simulink model "pospoli_XY_traiettoria"  (R2020b)
settings: Solver=ode15s  StartTime=0.0  StopTime=tsim  MaxStep=0.024  RelTol=1e-3
values from neighbouring files (symbols this model uses):
  Acc_asse_x = []    [Main_Strategia_di_pilotaggio.m]
  Acc_asse_y = []    [Main_Strategia_di_pilotaggio.m]
  mx = config_dc_x(parx)    [Main_Strategia_di_pilotaggio.m]    (also in Main_traiettoria.m; Main_traiettoria_ordinato.m)
  my = config_dc_y(pary)    [Main_Strategia_di_pilotaggio.m]    (also in Main_traiettoria.m; Main_traiettoria_ordinato.m)
  ppx_c = pos_poli_cc_x(mx, acx, 2)    [Main_Strategia_di_pilotaggio.m]
  ppx_m = pos_poli_cc_x(mx, acx, 1)    [Main_Strategia_di_pilotaggio.m]
  ppy_c = pos_poli_cc_y(my, acy, 2)    [Main_Strategia_di_pilotaggio.m]
  ppy_m = pos_poli_cc_y(my, acy, 1)    [Main_Strategia_di_pilotaggio.m]
  time = 0:tf/np:tf    [Main_traiettoria.m]    (also in Main_traiettoria_ordinato.m = 0:passo:tsim)
  Vel_asse_x = []    [Main_Strategia_di_pilotaggio.m]
  Vel_asse_y = []    [Main_Strategia_di_pilotaggio.m]
  x = []    [Main_Strategia_di_pilotaggio.m]    (also in Main_traiettoria.m = zeros(length(time),1); Main_traiettoria_ordinato.m = zeros(length(time),1); interpolazione_tempi.m = interp1(t_m,x_i,u,'Linear'))
  y = []    [Main_Strategia_di_pilotaggio.m]    (also in Main_traiettoria.m = zeros(length(time),1); Main_traiettoria_ordinato.m = zeros(length(time),1); interpolazione_tempi.m = interp1(t_m,y_i,u,'Linear'))
undefined symbols (not defined in the file or in its folder): accelerazioni, accelerazioniy, ci_x, ci_y, Evaluate_Trajectory, interpolazione_tempi, parx, pary
libraries: simulink x2
settings Model: Creator=stefa  LastModifiedBy=user
settings DebuggingCC: AlgebraicLoopMsg=none  SFMachineParentedDataDiag=error

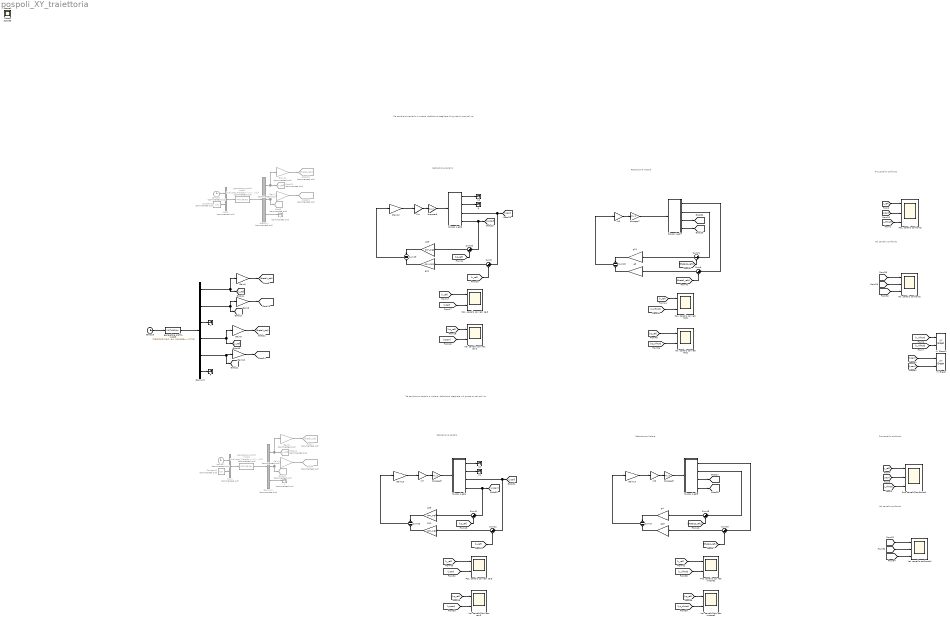
== system pospoli_XY_traiettoria ==
  note: Se cambiamo carrello o motore, dobbiamo scegliere w0 giusta su pos poli cc
  note: Retroazione Motore
  note: Se cambiamo carrello o motore, dobbiamo scegliere w0 giusta su pos poli cc
  note: Retroazione carrello
  note: Retroazione carrello
  note: Retroazione Motore
  note: Vel carrello confronto
  note: Pos carrello confronto
  note: Vel carrello confronto
  note: Pos carrello confronto
  " 1" : Terminator  Commented=on
   {7..12} (6 alike) : Terminator
  " 4" : Terminator  Commented=on
  Constant1 : Constant  Commented=on  Value=0.6
  Constant2 : Constant  Commented=on  Value=0.6
  Demux1 : Demux  Commented=on  Outputs=3
  Demux2 : Demux  Commented=on  Outputs=3
  Demux3 : Demux  Outputs=6
  Gain{9..10,13..14} (4 alike) : Gain  Gain=1/pary.tau
  Gain11 : Gain  Commented=on  Gain=1/parx.tau
  Gain12 : Gain  Gain=1/parx.tau
  Gain3 : Gain  Commented=on  Gain=1/pary.tau
  Gain4 : Gain  Commented=on  Gain=1/pary.tau
  Gain6 : Gain  Gain=1/parx.tau
  Gain7 : Gain  Commented=on  Gain=1/parx.tau
  Gain8 : Gain  Gain=1/parx.tau
  Goto10 : Goto  Commented=on  GotoTag=y_ref
  Goto11 : Goto  Commented=on  GotoTag=yp_ref
  Goto18 : Goto  Commented=on  GotoTag=theta1_refx
  Goto20 : Goto  Commented=on  GotoTag=theta1p_refx
  Goto23 : Goto  Commented=on  GotoTag=x_ref
  Goto5 : Goto  Commented=on  GotoTag=xp_ref
  Goto7 : Goto  Commented=on  GotoTag=theta1_refy
  Goto9 : Goto  Commented=on  GotoTag=theta1p_refy
  Kr4 : Gain  Gain=mx.Kr
  Kr6 : Gain  Gain=mx.Kr
  Kr7 : Gain  Gain=my.Kr
  Kr8 : Gain  Gain=my.Kr
  Mux1 : Mux  Commented=on  Inputs=2
  Mux2 : Mux  Commented=on  Inputs=2
  Pos. carrello con retr. Mot1 : Scope  NumInputPorts=2
  Pos. carrello con retr. car2 : Scope  NumInputPorts=2
  Pos. carrello con retr. car3 : Scope  NumInputPorts=2
  Pos. carrello con retr. motore1 : Scope  NumInputPorts=2
  Pos. carrello confronto : Scope  NumInputPorts=3
  Pos. carrello confronto1 : Scope  NumInputPorts=3
  Sum{6,8,11,15..16,20..22} (8 alike) : Sum  Inputs=|+-
  Sum{17..19,23} (4 alike) : Sum  Inputs=--
  Vel. carrello con retr. Mot1 : Scope  NumInputPorts=2
  Vel. carrello con retr. car.2 : Scope  NumInputPorts=2
  Vel. carrello con retr. car.3 : Scope  NumInputPorts=2
  Vel. carrello con retr. motore1 : Scope  NumInputPorts=2
  Vel. carrello confronto : Scope  NumInputPorts=3
  Vel. carrello confronto1 : Scope  NumInputPorts=3
  XY Graph : simulink/Sinks/XY Graph  xmin=-0.5  xmax=0.5  ymin=-0.5  ymax=0.5  st=-1
  XY Graph1 : simulink/Sinks/XY Graph  xmin=-0.5  xmax=0.5  ymin=-0.5  ymax=0.5  st=-1
  blocco 4 gdl4 : Subsystem
  blocco 4 gdl6 : Subsystem
  blocco 4 gdl7 : Subsystem
  blocco 4 gdl8 : Subsystem
  chopper3 : Gain  Gain=my.K
  chopper6 : Gain  Gain=mx.K
  chopper7 : Gain  Gain=mx.K
  chopper8 : Gain  Gain=my.K
  g11 : Gain  Gain=ppx_m.g2
  g12 : Gain  Gain=ppx_c.g1
  g13 : Gain  Gain=ppx_c.g2
  g14 : Gain  Gain=ppy_c.g1
  g15 : Gain  Gain=ppy_c.g2
  g16 : Gain  Gain=ppy_m.g1
  g3 : Gain  Gain=ppx_m.g1
  g4 : Gain  Gain=ppy_m.g2
  generatore profilo moto1 : MATLABFcn  Commented=on  MATLABFcn=Evaluate_Trajectory( u(1) , u(2))  OutputDimensions=3
  generatore profilo moto2 : MATLABFcn  Commented=on  MATLABFcn=Evaluate_Trajectory( u(1) , u(2))  OutputDimensions=3
  generatore profilo moto3 : MATLABFcn  MATLABFcn=interpolazione_tempi(x,Vel_asse_x,Acc_asse_x,y,Vel_asse_y,Acc_asse_y,u,time)
  tempo1 : Clock  Commented=on
  tempo2 : Clock  Commented=on
  tempo3 : Clock
      settings: Decimation=tsim
  Scope : Scope
  Scope1 : Scope
  Scope3 : Scope
  wires:
  Mux2/1 -> generatore profilo moto1/1
  Gain7/1 -> Goto20/1  "motore"
  Gain11/1 -> Goto18/1  "motore"
  Constant2/1 -> Mux2/2
  Demux1/3 -> " 1"/1  "XPP"
  tempo1/1 -> Mux2/1
  generatore profilo moto1/1 -> Demux1/1  "carrello"
  Demux1/2 -> Gain7/1, Goto5/1  "XP"
  Demux1/1 -> Goto23/1, Gain11/1  "X"
  tempo2/1 -> Mux1/1
  generatore profilo moto2/1 -> Demux2/1  "carrello"
  Demux2/2 -> Gain4/1, Goto11/1  "YP"
  Constant1/1 -> Mux1/2
  Mux1/1 -> generatore profilo moto2/1
  Gain4/1 -> Goto9/1  "motore"
  Gain3/1 -> Goto7/1  "motore"
  Demux2/1 -> Goto10/1, Gain3/1  "Y"
  Demux2/3 -> " 4"/1  "YPP"
  generatore profilo moto3/1 -> Demux3/1  "carrello"
  tempo3/1 -> generatore profilo moto3/1
  Demux3/6 -> " 8"/1  "YPP"
  Gain6/1 -> [theta1_refx]  "motore"
  Demux3/3 -> " 7"/1  "XPP"
  Demux3/1 -> [x_ref], Gain6/1  "X"
  Demux3/2 -> Gain8/1, [xp_ref]  "XP"
  Gain8/1 -> [theta1p_refx]  "motore"
  Gain9/1 -> [theta1_refy]  "motore"
  Gain10/1 -> [theta1p_refy]  "motore"
  Demux3/4 -> [y_ref], Gain9/1  "Y"
  Demux3/5 -> [yp_ref], Gain10/1  "YP"
  [x_rifmot] -> Pos. carrello con retr. Mot1/2  "motore"
  Kr7/1 -> chopper3/1  "I"
  Sum21/1 -> g11/1
  [theta1p_refx] -> Sum21/2
  Sum20/1 -> g13/1
  blocco 4 gdl7/1(Out3) -> Sum6/1
  g12/1 -> Sum19/2  "Cm"
  chopper6/1 -> blocco 4 gdl6/1(In1)  "Cm"
  chopper7/1 -> blocco 4 gdl7/1(In1)  "Cm"
  Sum6/1 -> g3/1
  g3/1 -> Sum18/2  "Cm"
  Sum18/1 -> Kr6/1  "Va"
  blocco 4 gdl7/4(Out1) -> [xp_rifmot]
  Kr6/1 -> chopper7/1  "I"
  g11/1 -> Sum18/1  "Cm"
  blocco 4 gdl8/4(Out1) -> [yp_rifmot]
  Gain14/1 -> Kr8/1  "motore"
  Sum16/1 -> g16/1
  blocco 4 gdl8/3(Out3) -> [y_rifmot]
  g4/1 -> Sum17/1  "Cm"
  [xcarr] -> Pos. carrello con retr. car2/2  "carrello"
  g15/1 -> Sum23/1  "Cm"
  Sum15/1 -> g4/1
  Kr8/1 -> chopper8/1  "I"
  blocco 4 gdl8/1(Out2) -> Sum16/1
  [theta1_refy] -> Sum16/2
  [yp_ref] -> Vel. carrello con retr. car.3/1
  g13/1 -> Sum19/1  "Cm"
  [theta1_refx] -> Sum6/2
  g14/1 -> Sum23/2  "Cm"
  blocco 4 gdl8/2(Out5) -> Sum15/1
  blocco 4 gdl4/3(Out3) -> Sum22/1, [ycarr]
  blocco 4 gdl6/1(Out3) -> " 10"/1
  [y_ref] -> Pos. carrello con retr. car3/1
  [x_ref] -> Sum8/2
  g16/1 -> Sum17/2  "Cm"
  blocco 4 gdl4/2(Out5) -> " 11"/1
  Sum22/1 -> g14/1
  blocco 4 gdl4/1(Out2) -> " 12"/1
  Kr4/1 -> chopper6/1  "I"
  blocco 4 gdl7/2(Out4) -> Sum21/1
  [xp_ref] -> Vel. carrello con retr. car.2/1
  Sum19/1 -> Gain12/1
  [yp_ref] -> Sum11/2
  blocco 4 gdl6/3(Out7) -> Sum8/1, [xcarr]
  blocco 4 gdl4/4(Out1) -> Sum11/1, [ypcarr]
  blocco 4 gdl6/2(Out4) -> " 9"/1
  Sum17/1 -> Gain14/1
  [ycarr] -> Pos. carrello con retr. car3/2  "carrello"
  [yp_ref] -> Vel. carrello con retr. motore1/1
  [x_ref] -> Pos. carrello con retr. car2/1
  chopper8/1 -> blocco 4 gdl8/1(In2)  "Cm"
  chopper3/1 -> blocco 4 gdl4/1(In2)  "Cm"
  Gain12/1 -> Kr4/1  "motore"
  [y_ref] -> Sum22/2
  [x_ref] -> Pos. carrello con retr. Mot1/1
  [xp_ref] -> Vel. carrello con retr. Mot1/1
  Sum23/1 -> Gain13/1
  [xp_rifmot] -> Vel. carrello con retr. Mot1/2  "motore"
  blocco 4 gdl7/3(Out7) -> [x_rifmot]
  [yp_rifmot] -> Vel. carrello con retr. motore1/2  "carrello"
  [theta1p_refy] -> Sum15/2
  blocco 4 gdl6/4(Out1) -> Sum20/1, [xpcarr]
  [xpcarr] -> Vel. carrello con retr. car.2/2  "carrello"
  [y_rifmot] -> Pos. carrello con retr. motore1/2  "carrello"
  [ypcarr] -> Vel. carrello con retr. car.3/2  "carrello"
  Gain13/1 -> Kr7/1  "motore"
  Sum8/1 -> g12/1
  [xp_ref] -> Sum20/2
  [y_ref] -> Pos. carrello con retr. motore1/1
  Sum11/1 -> g15/1
  [y_rifmot] -> Pos. carrello confronto1/3  "y retr. motore"
  [xcarr] -> Pos. carrello confronto/2  "x_retcarr"
  [ypcarr] -> Vel. carrello confronto1/2  "yp retr. carrello"
  [xcarr] -> XY Graph/1  "x_retcarr"
  [x_rifmot] -> Pos. carrello confronto/3  "x_retmot"
  [xp_rifmot] -> Vel. carrello confronto/3  "xp_retmot"
  [ycarr] -> Pos. carrello confronto1/2  "y retr. carrello"
  [yp_rifmot] -> Vel. carrello confronto1/3  "yp retr. motore"
  [xp_ref] -> Vel. carrello confronto/1  "xp_ref"
  [x_ref] -> Pos. carrello confronto/1  "x_ref"
  [yp_ref] -> Vel. carrello confronto1/1  "yp ldm"
  [y_ref] -> Pos. carrello confronto1/1  "y ldm"
  [xpcarr] -> Vel. carrello confronto/2  "xp_retcarr"
  [ycarr] -> XY Graph/2  "y retr. carrello"
  [x_rifmot] -> XY Graph1/1  "motore"
  [y_rifmot] -> XY Graph1/2  "motore"

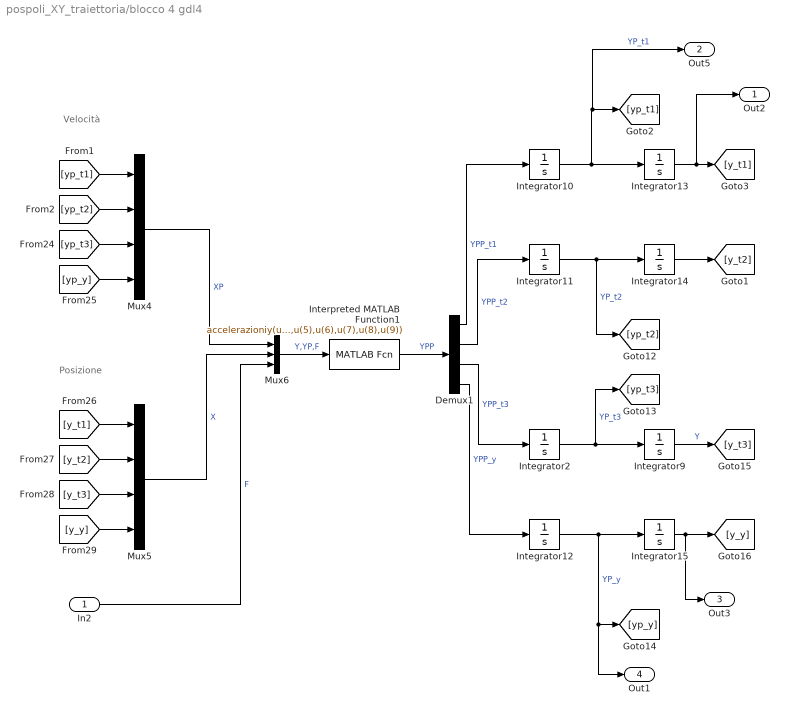
== system pospoli_XY_traiettoria/blocco 4 gdl4 ==
  note: Posizione
  note: Velocità
  In2 : Inport
  Demux1 : Demux
  Integrator{2,10..12} (4 alike) : Integrator
  Integrator13 : Integrator  InitialCondition=ci_y(1)
  Integrator14 : Integrator  InitialCondition=ci_y(2)
  Integrator15 : Integrator  InitialCondition=ci_y(4)
  Integrator9 : Integrator  InitialCondition=ci_y(3)
  Interpreted MATLAB Function1 : MATLABFcn  MATLABFcn=accelerazioniy(u(1),u(2),u(3),u(4),u(5),u(6),u(7),u(8),u(9))  OutputDimensions=4
  Mux4 : Mux
  Mux5 : Mux
  Mux6 : Mux  Inputs=3
  Out2 : Outport
  Out5 : Outport  Port=2
  Out3 : Outport  Port=3
  Out1 : Outport  Port=4
  wires:
  Mux4/1 -> Mux6/1  "XP"
  Integrator9/1 -> [y_t3]  "Y"
  [y_t2] -> Mux5/2
  [yp_t1] -> Mux4/1
  Integrator13/1 -> Out2/1, [y_t1]
  Demux1/4 -> Integrator12/1  "YPP_y"
  Integrator12/1 -> Out1/1, [yp_y], Integrator15/1  "YP_y"
  [yp_t3] -> Mux4/3
  Integrator2/1 -> [yp_t3], Integrator9/1  "YP_t3"
  Integrator11/1 -> [yp_t2], Integrator14/1  "YP_t2"
  Demux1/1 -> Integrator10/1  "YPP_t1"
  Integrator10/1 -> Out5/1, [yp_t1], Integrator13/1  "YP_t1"
  [y_t1] -> Mux5/1
  Mux5/1 -> Mux6/2  "X"
  [y_t3] -> Mux5/3
  Demux1/2 -> Integrator11/1  "YPP_t2"
  Interpreted MATLAB Function1/1 -> Demux1/1  "YPP"
  [yp_t2] -> Mux4/2
  [yp_y] -> Mux4/4
  Integrator14/1 -> [y_t2]
  Integrator15/1 -> Out3/1, [y_y]
  Demux1/3 -> Integrator2/1  "YPP_t3"
  Mux6/1 -> Interpreted MATLAB Function1/1  "Y,YP,F"
  [y_y] -> Mux5/4
  In2/1 -> Mux6/3  "F"

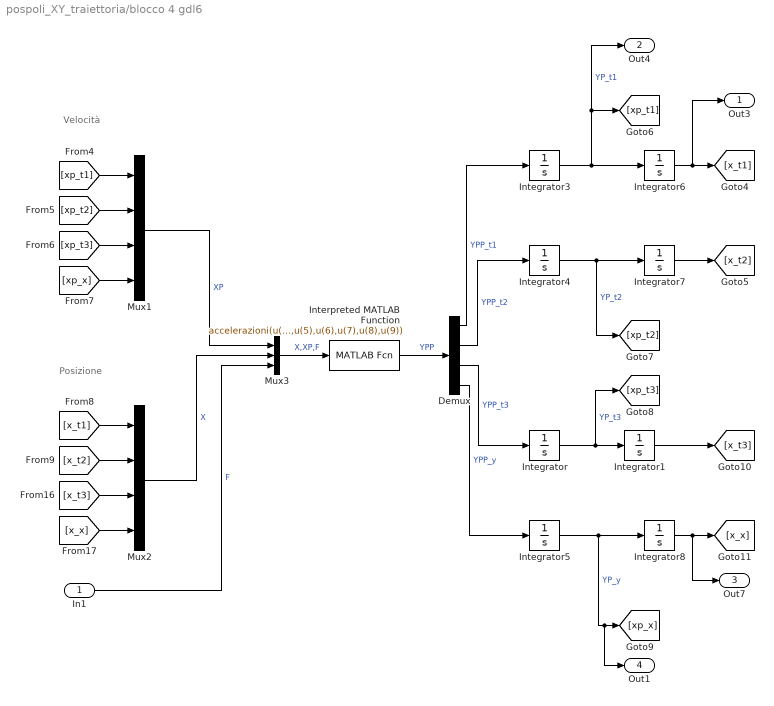
== system pospoli_XY_traiettoria/blocco 4 gdl6 ==
  note: Posizione
  note: Velocità
  In1 : Inport
  Demux : Demux
  Integrator{,3..5} (4 alike) : Integrator
  Integrator1 : Integrator  InitialCondition=ci_x(3)
  Integrator6 : Integrator  InitialCondition=ci_x(1)
  Integrator7 : Integrator  InitialCondition=ci_x(2)
  Integrator8 : Integrator  InitialCondition=ci_x(4)
  Interpreted MATLAB Function : MATLABFcn  MATLABFcn=accelerazioni(u(1),u(2),u(3),u(4),u(5),u(6),u(7),u(8),u(9))  OutputDimensions=4
  Mux1 : Mux
  Mux2 : Mux
  Mux3 : Mux  Inputs=3
  Out3 : Outport
  Out4 : Outport  Port=2
  Out7 : Outport  Port=3
  Out1 : Outport  Port=4
  wires:
  [xp_t3] -> Mux1/3
  Interpreted MATLAB Function/1 -> Demux/1  "YPP"
  Integrator3/1 -> Out4/1, [xp_t1], Integrator6/1  "YP_t1"
  Integrator8/1 -> Out7/1, [x_x]
  Integrator7/1 -> [x_t2]
  [xp_x] -> Mux1/4
  [x_t1] -> Mux2/1
  Mux1/1 -> Mux3/1  "XP"
  [x_x] -> Mux2/4
  Demux/3 -> Integrator/1  "YPP_t3"
  Integrator/1 -> Integrator1/1, [xp_t3]  "YP_t3"
  Mux2/1 -> Mux3/2  "X"
  Integrator6/1 -> Out3/1, [x_t1]
  Integrator5/1 -> Out1/1, [xp_x], Integrator8/1  "YP_y"
  [xp_t2] -> Mux1/2
  Mux3/1 -> Interpreted MATLAB Function/1  "X,XP,F"
  [x_t3] -> Mux2/3
  In1/1 -> Mux3/3  "F"
  Demux/4 -> Integrator5/1  "YPP_y"
  Integrator4/1 -> [xp_t2], Integrator7/1  "YP_t2"
  Integrator1/1 -> [x_t3]
  [xp_t1] -> Mux1/1
  [x_t2] -> Mux2/2
  Demux/2 -> Integrator4/1  "YPP_t2"
  Demux/1 -> Integrator3/1  "YPP_t1"

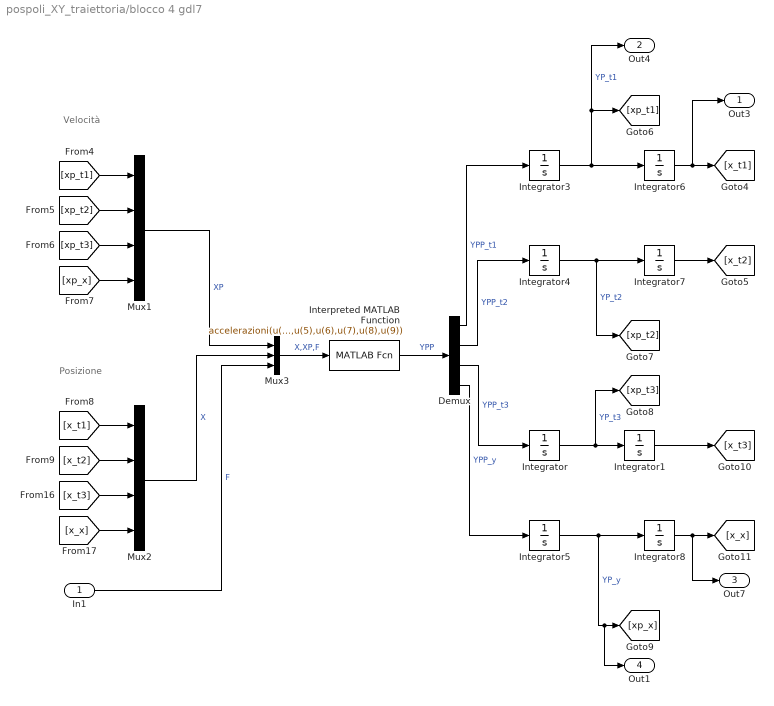
== system pospoli_XY_traiettoria/blocco 4 gdl7 ==
  note: Posizione
  note: Velocità
  In1 : Inport
  Demux : Demux
  Integrator{,3..5} (4 alike) : Integrator
  Integrator1 : Integrator  InitialCondition=ci_x(3)
  Integrator6 : Integrator  InitialCondition=ci_x(1)
  Integrator7 : Integrator  InitialCondition=ci_x(2)
  Integrator8 : Integrator  InitialCondition=ci_x(4)
  Interpreted MATLAB Function : MATLABFcn  MATLABFcn=accelerazioni(u(1),u(2),u(3),u(4),u(5),u(6),u(7),u(8),u(9))  OutputDimensions=4
  Mux1 : Mux
  Mux2 : Mux
  Mux3 : Mux  Inputs=3
  Out3 : Outport
  Out4 : Outport  Port=2
  Out7 : Outport  Port=3
  Out1 : Outport  Port=4
  wires:
  [xp_t3] -> Mux1/3
  Interpreted MATLAB Function/1 -> Demux/1  "YPP"
  Integrator3/1 -> Out4/1, [xp_t1], Integrator6/1  "YP_t1"
  Integrator8/1 -> Out7/1, [x_x]
  Integrator7/1 -> [x_t2]
  [xp_x] -> Mux1/4
  [x_t1] -> Mux2/1
  Mux1/1 -> Mux3/1  "XP"
  [x_x] -> Mux2/4
  Demux/3 -> Integrator/1  "YPP_t3"
  Integrator/1 -> Integrator1/1, [xp_t3]  "YP_t3"
  Mux2/1 -> Mux3/2  "X"
  Integrator6/1 -> Out3/1, [x_t1]
  Integrator5/1 -> Out1/1, [xp_x], Integrator8/1  "YP_y"
  [xp_t2] -> Mux1/2
  Mux3/1 -> Interpreted MATLAB Function/1  "X,XP,F"
  [x_t3] -> Mux2/3
  In1/1 -> Mux3/3  "F"
  Demux/4 -> Integrator5/1  "YPP_y"
  Integrator4/1 -> [xp_t2], Integrator7/1  "YP_t2"
  Integrator1/1 -> [x_t3]
  [xp_t1] -> Mux1/1
  [x_t2] -> Mux2/2
  Demux/2 -> Integrator4/1  "YPP_t2"
  Demux/1 -> Integrator3/1  "YPP_t1"

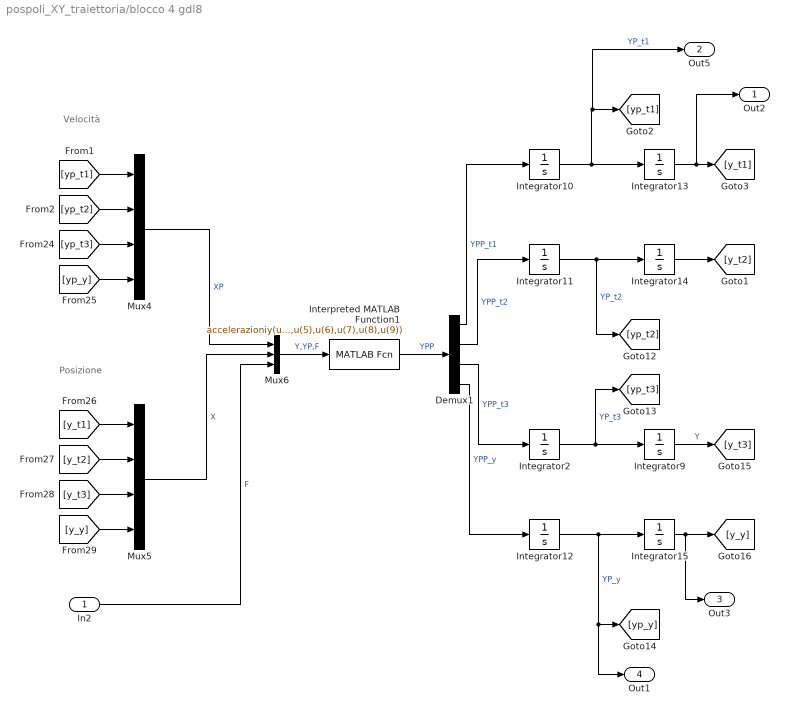
== system pospoli_XY_traiettoria/blocco 4 gdl8 ==
  note: Posizione
  note: Velocità
  In2 : Inport
  Demux1 : Demux
  Integrator{2,10..12} (4 alike) : Integrator
  Integrator13 : Integrator  InitialCondition=ci_y(1)
  Integrator14 : Integrator  InitialCondition=ci_y(2)
  Integrator15 : Integrator  InitialCondition=ci_y(4)
  Integrator9 : Integrator  InitialCondition=ci_y(3)
  Interpreted MATLAB Function1 : MATLABFcn  MATLABFcn=accelerazioniy(u(1),u(2),u(3),u(4),u(5),u(6),u(7),u(8),u(9))  OutputDimensions=4
  Mux4 : Mux
  Mux5 : Mux
  Mux6 : Mux  Inputs=3
  Out2 : Outport
  Out5 : Outport  Port=2
  Out3 : Outport  Port=3
  Out1 : Outport  Port=4
  wires:
  Mux4/1 -> Mux6/1  "XP"
  Integrator9/1 -> [y_t3]  "Y"
  [y_t2] -> Mux5/2
  [yp_t1] -> Mux4/1
  Integrator13/1 -> Out2/1, [y_t1]
  Demux1/4 -> Integrator12/1  "YPP_y"
  Integrator12/1 -> Out1/1, [yp_y], Integrator15/1  "YP_y"
  [yp_t3] -> Mux4/3
  Integrator2/1 -> [yp_t3], Integrator9/1  "YP_t3"
  Integrator11/1 -> [yp_t2], Integrator14/1  "YP_t2"
  Demux1/1 -> Integrator10/1  "YPP_t1"
  Integrator10/1 -> Out5/1, [yp_t1], Integrator13/1  "YP_t1"
  [y_t1] -> Mux5/1
  Mux5/1 -> Mux6/2  "X"
  [y_t3] -> Mux5/3
  Demux1/2 -> Integrator11/1  "YPP_t2"
  Interpreted MATLAB Function1/1 -> Demux1/1  "YPP"
  [yp_t2] -> Mux4/2
  [yp_y] -> Mux4/4
  Integrator14/1 -> [y_t2]
  Integrator15/1 -> Out3/1, [y_y]
  Demux1/3 -> Integrator2/1  "YPP_t3"
  Mux6/1 -> Interpreted MATLAB Function1/1  "Y,YP,F"
  [y_y] -> Mux5/4
  In2/1 -> Mux6/3  "F"
